simulink model "Control_Logic_a"  (R2018b)
settings: Solver=VariableStepAuto  StartTime=Start_time  StopTime=Stop_time  RelTol=1e-3
values from neighbouring files (symbols this model uses):
  Aset_N1 = 2    [Parameter_control.m]
  Aset_N10 = -10    [Parameter_control.m]
  Aset_N11 = 10    [Parameter_control.m]
  Aset_N12 = 20    [Parameter_control.m]
  Aset_N13 = 20    [Parameter_control.m]
  Aset_N2 = 30    [Parameter_control.m]
  Aset_N3 = 3    [Parameter_control.m]
  Aset_N4 = 5    [Parameter_control.m]
  Aset_N5 = 1    [Parameter_control.m]
  Aset_N6 = 0    [Parameter_control.m]
  Aset_N7 = 0.01    [Parameter_control.m]
  Aset_N8 = 2    [Parameter_control.m]
  Aset_N9 = 0.1    [Parameter_control.m]
  Dset_N1 = 1    [Parameter_control.m]
  Dset_N2 = 1    [Parameter_control.m]
  Ini_time = Start_time    (= 0)    [main.m]
  Sample_time = 0.1    [main.m]    (also in manual_env_for_test_slx.m; test_tool_initialize.m)
undefined symbols (not defined in the file or in its folder): DiscIntNeverNeededParam
(part 2 of 2)

== system Control_Logic_a/OST7 ==
  In : Inport  OutDataTypeStr=boolean  SampleTime=Sample_time
  T : Inport  Port=2  OutDataTypeStr=double  SampleTime=Sample_time
  Add : Sum  OutDataTypeStr=double
  Constant1 : Constant  SampleTime=Sample_time
  Discrete-Time Integrator1 : DiscreteIntegrator  SampleTime=Sample_time  LimitOutput=on  LowerSaturationLimit=0  ICPrevOutput=DiscIntNeverNeededParam  ICPrevScaledInput=DiscIntNeverNeededParam
  Logical Operator1 : Logic  AllPortsSameDT=off  OutDataTypeStr=boolean
  Max : MinMax  Inputs=2  OutDataTypeStr=double
  Parameter : Constant  Value=0  OutDataTypeStr=double  SampleTime=Sample_time
  Relational Operator : RelationalOperator  Operator=>  OutDataTypeStr=boolean  RndMeth=Nearest
  Sub : Sum  Inputs=+-  AccumDataTypeStr=single  OutDataTypeStr=double
  Switch : Switch  Criteria=u2 > Threshold  Threshold=0.5  OutDataTypeStr=double
  Unit Delay : UnitDelay  SampleTime=Sample_time
  Unit Delay2 : UnitDelay  InitialCondition=Ini_time  SampleTime=Sample_time
  Out : Outport  OutDataTypeStr=boolean  SampleTime=Sample_time
  wires:
  Constant1/1 -> Discrete-Time Integrator1/1
  Max/1 -> Relational Operator/2, Unit Delay/1
  T/1 -> Max/1, Relational Operator/1
  Add/1 -> Max/2
  Parameter/1 -> Switch/3
  Unit Delay/1 -> Switch/1
  Switch/1 -> Add/2
  Relational Operator/1 -> Logical Operator1/1
  Logical Operator1/1 -> Out/1
  Sub/1 -> Add/1
  Unit Delay2/1 -> Sub/2
  Discrete-Time Integrator1/1 -> Sub/1, Unit Delay2/1
  In/1 -> Logical Operator1/2, Switch/2

== system Control_Logic_a/OST8 ==
  In : Inport  OutDataTypeStr=boolean  SampleTime=Sample_time
  T : Inport  Port=2  OutDataTypeStr=double  SampleTime=Sample_time
  Add : Sum  OutDataTypeStr=double
  Constant1 : Constant  SampleTime=Sample_time
  Discrete-Time Integrator1 : DiscreteIntegrator  SampleTime=Sample_time  LimitOutput=on  LowerSaturationLimit=0  ICPrevOutput=DiscIntNeverNeededParam  ICPrevScaledInput=DiscIntNeverNeededParam
  Logical Operator1 : Logic  AllPortsSameDT=off  OutDataTypeStr=boolean
  Max : MinMax  Inputs=2  OutDataTypeStr=double
  Parameter : Constant  Value=0  OutDataTypeStr=double  SampleTime=Sample_time
  Relational Operator : RelationalOperator  Operator=>  OutDataTypeStr=boolean  RndMeth=Nearest
  Sub : Sum  Inputs=+-  AccumDataTypeStr=single  OutDataTypeStr=double
  Switch : Switch  Criteria=u2 > Threshold  Threshold=0.5  OutDataTypeStr=double
  Unit Delay : UnitDelay  SampleTime=Sample_time
  Unit Delay2 : UnitDelay  InitialCondition=Ini_time  SampleTime=Sample_time
  Out : Outport  OutDataTypeStr=boolean  SampleTime=Sample_time
  wires:
  Constant1/1 -> Discrete-Time Integrator1/1
  Max/1 -> Relational Operator/2, Unit Delay/1
  T/1 -> Max/1, Relational Operator/1
  Add/1 -> Max/2
  Parameter/1 -> Switch/3
  Unit Delay/1 -> Switch/1
  Switch/1 -> Add/2
  Relational Operator/1 -> Logical Operator1/1
  Logical Operator1/1 -> Out/1
  Sub/1 -> Add/1
  Unit Delay2/1 -> Sub/2
  Discrete-Time Integrator1/1 -> Sub/1, Unit Delay2/1
  In/1 -> Logical Operator1/2, Switch/2

== system Control_Logic_a/OST9 ==
  In : Inport  OutDataTypeStr=boolean  SampleTime=Sample_time
  T : Inport  Port=2  OutDataTypeStr=double  SampleTime=Sample_time
  Add : Sum  OutDataTypeStr=double
  Constant1 : Constant  SampleTime=Sample_time
  Discrete-Time Integrator1 : DiscreteIntegrator  SampleTime=Sample_time  LimitOutput=on  LowerSaturationLimit=0  ICPrevOutput=DiscIntNeverNeededParam  ICPrevScaledInput=DiscIntNeverNeededParam
  Logical Operator1 : Logic  AllPortsSameDT=off  OutDataTypeStr=boolean
  Max : MinMax  Inputs=2  OutDataTypeStr=double
  Parameter : Constant  Value=0  OutDataTypeStr=double  SampleTime=Sample_time
  Relational Operator : RelationalOperator  Operator=>  OutDataTypeStr=boolean  RndMeth=Nearest
  Sub : Sum  Inputs=+-  AccumDataTypeStr=single  OutDataTypeStr=double
  Switch : Switch  Criteria=u2 > Threshold  Threshold=0.5  OutDataTypeStr=double
  Unit Delay : UnitDelay  SampleTime=Sample_time
  Unit Delay2 : UnitDelay  InitialCondition=Ini_time  SampleTime=Sample_time
  Out : Outport  OutDataTypeStr=boolean  SampleTime=Sample_time
  wires:
  Constant1/1 -> Discrete-Time Integrator1/1
  In/1 -> Switch/2, Logical Operator1/2
  Discrete-Time Integrator1/1 -> Unit Delay2/1, Sub/1
  Unit Delay2/1 -> Sub/2
  Sub/1 -> Add/1
  Logical Operator1/1 -> Out/1
  Relational Operator/1 -> Logical Operator1/1
  Switch/1 -> Add/2
  Unit Delay/1 -> Switch/1
  Parameter/1 -> Switch/3
  Add/1 -> Max/2
  T/1 -> Relational Operator/1, Max/1
  Max/1 -> Unit Delay/1, Relational Operator/2

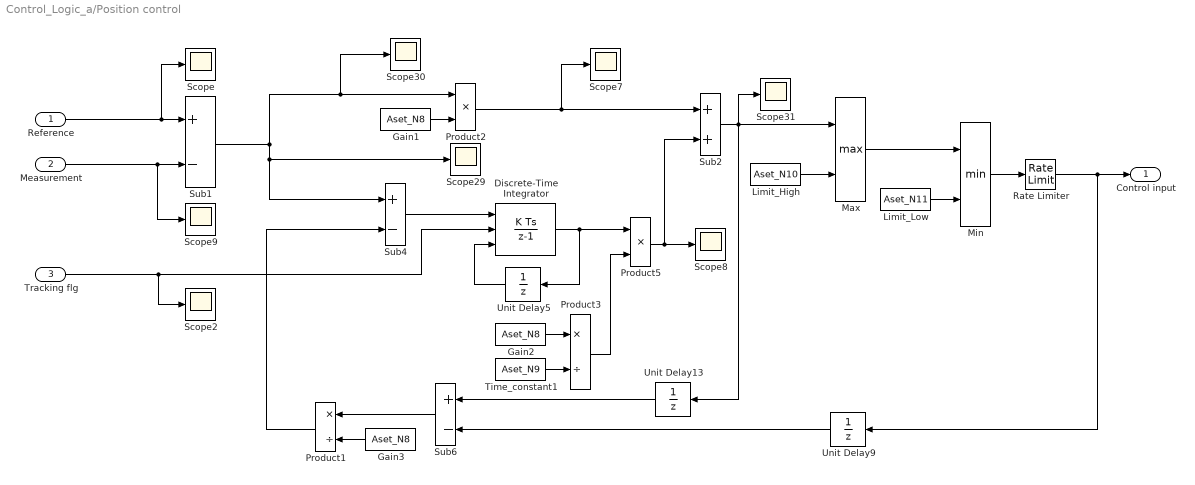
== system Control_Logic_a/Position control ==
  Reference : Inport
  Measurement : Inport  Port=2
  Tracking flg : Inport  Port=3
  Discrete-Time Integrator : DiscreteIntegrator  ExternalReset=level  InitialConditionSource=external  SampleTime=Sample_time  ICPrevOutput=DiscIntNeverNeededParam  ICPrevScaledInput=DiscIntNeverNeededParam
  Gain1 : Constant  Value=Aset_N8  OutDataTypeStr=double  SampleTime=Sample_time
  Gain2 : Constant  Value=Aset_N8  OutDataTypeStr=double  SampleTime=Sample_time
  Gain3 : Constant  Value=Aset_N8  OutDataTypeStr=double  SampleTime=Sample_time
  Limit_High : Constant  Value=Aset_N10  OutDataTypeStr=double  SampleTime=Sample_time
  Limit_Low : Constant  Value=Aset_N11  OutDataTypeStr=double  SampleTime=Sample_time
  Max : MinMax  Function=max  Inputs=2
  Min : MinMax  Inputs=2
  Product1 : Product  Inputs=*/  OutDataTypeStr=double  RndMeth=Zero
  Product2 : Product  OutDataTypeStr=double  RndMeth=Zero
  Product3 : Product  Inputs=*/  OutDataTypeStr=double  RndMeth=Zero
  Product5 : Product  Inputs=**  OutDataTypeStr=double  RndMeth=Zero
  Rate Limiter : RateLimiter  RisingSlewLimit=Aset_N12  FallingSlewLimit=-1*Aset_N13  SampleTimeMode=inherited
  Scope{,2,7..9,29..31} (8 alike) : Scope
  Sub1 : Sum  Inputs=+-  OutDataTypeStr=double
  Sub2 : Sum  OutDataTypeStr=double
  Sub4 : Sum  Inputs=+-  OutDataTypeStr=double
  Sub6 : Sum  Inputs=+-  OutDataTypeStr=double
  Time_constant1 : Constant  Value=Aset_N9  OutDataTypeStr=double  SampleTime=Sample_time
  Unit Delay13 : UnitDelay  SampleTime=Sample_time
  Unit Delay5 : UnitDelay  SampleTime=Sample_time
  Unit Delay9 : UnitDelay  SampleTime=Sample_time
  Control input : Outport
  wires:
  Sub2/1 -> Unit Delay13/1, Scope31/1, Max/1
  Measurement/1 -> Scope9/1, Sub1/2
  Sub1/1 -> Scope30/1, Product2/1, Scope29/1, Sub4/1
  Product3/1 -> Product5/2
  Unit Delay13/1 -> Sub6/1
  Product2/1 -> Scope7/1, Sub2/1
  Sub6/1 -> Product1/1
  Sub4/1 -> Discrete-Time Integrator/1
  Gain1/1 -> Product2/2
  Min/1 -> Rate Limiter/1
  Reference/1 -> Scope/1, Sub1/1
  Gain3/1 -> Product1/2
  Limit_Low/1 -> Min/2
  Unit Delay5/1 -> Discrete-Time Integrator/3
  Tracking flg/1 -> Scope2/1, Discrete-Time Integrator/2
  Discrete-Time Integrator/1 -> Unit Delay5/1, Product5/1
  Limit_High/1 -> Max/2
  Product5/1 -> Scope8/1, Sub2/2
  Rate Limiter/1 -> Control input/1, Unit Delay9/1
  Time_constant1/1 -> Product3/2
  Gain2/1 -> Product3/1
  Max/1 -> Min/1
  Product1/1 -> Sub4/2
  Unit Delay9/1 -> Sub6/2

== system Control_Logic_a/SSR ==
  S : Inport
  R : Inport  Port=2
  Logical Operator1 : Logic  Operator=OR  AllPortsSameDT=off  OutDataTypeStr=boolean
  Logical Operator2 : Logic  AllPortsSameDT=off  OutDataTypeStr=boolean
  Logical Operator5 : Logic  Operator=NOT  AllPortsSameDT=off  OutDataTypeStr=boolean
  Unit Delay : UnitDelay  SampleTime=Sample_time
  Out : Outport
  wires:
  Logical Operator5/1 -> Logical Operator2/1
  R/1 -> Logical Operator5/1
  Unit Delay/1 -> Logical Operator2/2
  Logical Operator2/1 -> Logical Operator1/2
  Logical Operator1/1 -> Unit Delay/1, Out/1
  S/1 -> Logical Operator1/1

== system Control_Logic_a/SSR1 ==
  S : Inport
  R : Inport  Port=2
  Logical Operator1 : Logic  Operator=OR  AllPortsSameDT=off  OutDataTypeStr=boolean
  Logical Operator2 : Logic  AllPortsSameDT=off  OutDataTypeStr=boolean
  Logical Operator5 : Logic  Operator=NOT  AllPortsSameDT=off  OutDataTypeStr=boolean
  Unit Delay : UnitDelay  SampleTime=Sample_time
  Out : Outport
  wires:
  Logical Operator5/1 -> Logical Operator2/1
  R/1 -> Logical Operator5/1
  Unit Delay/1 -> Logical Operator2/2
  Logical Operator2/1 -> Logical Operator1/2
  Logical Operator1/1 -> Unit Delay/1, Out/1
  S/1 -> Logical Operator1/1

== system Control_Logic_a/SSR2 ==
  S : Inport
  R : Inport  Port=2
  Logical Operator1 : Logic  Operator=OR  AllPortsSameDT=off  OutDataTypeStr=boolean
  Logical Operator2 : Logic  AllPortsSameDT=off  OutDataTypeStr=boolean
  Logical Operator5 : Logic  Operator=NOT  AllPortsSameDT=off  OutDataTypeStr=boolean
  Unit Delay : UnitDelay  SampleTime=Sample_time
  Out : Outport
  wires:
  S/1 -> Logical Operator1/1
  Logical Operator1/1 -> Out/1, Unit Delay/1
  Logical Operator2/1 -> Logical Operator1/2
  Unit Delay/1 -> Logical Operator2/2
  R/1 -> Logical Operator5/1
  Logical Operator5/1 -> Logical Operator2/1

== system Control_Logic_a/SSR3 ==
  S : Inport
  R : Inport  Port=2
  Logical Operator1 : Logic  Operator=OR  AllPortsSameDT=off  OutDataTypeStr=boolean
  Logical Operator2 : Logic  AllPortsSameDT=off  OutDataTypeStr=boolean
  Logical Operator5 : Logic  Operator=NOT  AllPortsSameDT=off  OutDataTypeStr=boolean
  Unit Delay : UnitDelay  SampleTime=Sample_time
  Out : Outport
  wires:
  Logical Operator5/1 -> Logical Operator2/1
  R/1 -> Logical Operator5/1
  Unit Delay/1 -> Logical Operator2/2
  Logical Operator2/1 -> Logical Operator1/2
  Logical Operator1/1 -> Unit Delay/1, Out/1
  S/1 -> Logical Operator1/1

== system Control_Logic_a/SSR4 ==
  S : Inport
  R : Inport  Port=2
  Logical Operator1 : Logic  Operator=OR  AllPortsSameDT=off  OutDataTypeStr=boolean
  Logical Operator2 : Logic  AllPortsSameDT=off  OutDataTypeStr=boolean
  Logical Operator5 : Logic  Operator=NOT  AllPortsSameDT=off  OutDataTypeStr=boolean
  Unit Delay : UnitDelay  SampleTime=Sample_time
  Out : Outport
  wires:
  S/1 -> Logical Operator1/1
  Logical Operator1/1 -> Out/1, Unit Delay/1
  Logical Operator2/1 -> Logical Operator1/2
  Unit Delay/1 -> Logical Operator2/2
  R/1 -> Logical Operator5/1
  Logical Operator5/1 -> Logical Operator2/1

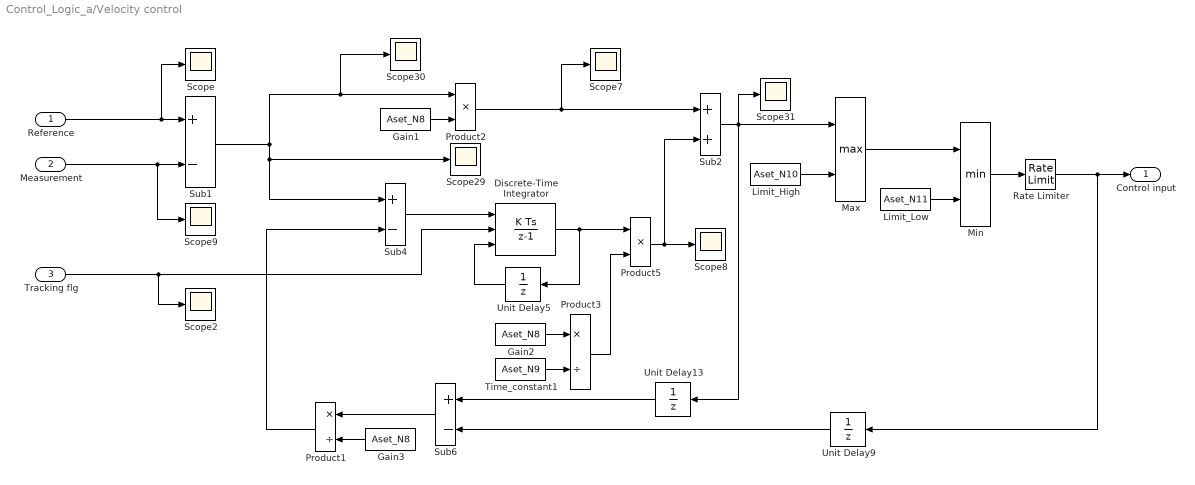
== system Control_Logic_a/Velocity control ==
  Reference : Inport
  Measurement : Inport  Port=2
  Tracking flg : Inport  Port=3
  Discrete-Time Integrator : DiscreteIntegrator  ExternalReset=level  InitialConditionSource=external  SampleTime=Sample_time  ICPrevOutput=DiscIntNeverNeededParam  ICPrevScaledInput=DiscIntNeverNeededParam
  Gain1 : Constant  Value=Aset_N8  OutDataTypeStr=double  SampleTime=Sample_time
  Gain2 : Constant  Value=Aset_N8  OutDataTypeStr=double  SampleTime=Sample_time
  Gain3 : Constant  Value=Aset_N8  OutDataTypeStr=double  SampleTime=Sample_time
  Limit_High : Constant  Value=Aset_N10  OutDataTypeStr=double  SampleTime=Sample_time
  Limit_Low : Constant  Value=Aset_N11  OutDataTypeStr=double  SampleTime=Sample_time
  Max : MinMax  Function=max  Inputs=2
  Min : MinMax  Inputs=2
  Product1 : Product  Inputs=*/  OutDataTypeStr=double  RndMeth=Zero
  Product2 : Product  OutDataTypeStr=double  RndMeth=Zero
  Product3 : Product  Inputs=*/  OutDataTypeStr=double  RndMeth=Zero
  Product5 : Product  Inputs=**  OutDataTypeStr=double  RndMeth=Zero
  Rate Limiter : RateLimiter  RisingSlewLimit=Aset_N12  FallingSlewLimit=-1*Aset_N13  SampleTimeMode=inherited
  Scope{,2,7..9,29..31} (8 alike) : Scope
  Sub1 : Sum  Inputs=+-  OutDataTypeStr=double
  Sub2 : Sum  OutDataTypeStr=double
  Sub4 : Sum  Inputs=+-  OutDataTypeStr=double
  Sub6 : Sum  Inputs=+-  OutDataTypeStr=double
  Time_constant1 : Constant  Value=Aset_N9  OutDataTypeStr=double  SampleTime=Sample_time
  Unit Delay13 : UnitDelay  SampleTime=Sample_time
  Unit Delay5 : UnitDelay  SampleTime=Sample_time
  Unit Delay9 : UnitDelay  SampleTime=Sample_time
  Control input : Outport
  wires:
  Unit Delay9/1 -> Sub6/2
  Product1/1 -> Sub4/2
  Max/1 -> Min/1
  Gain2/1 -> Product3/1
  Time_constant1/1 -> Product3/2
  Rate Limiter/1 -> Unit Delay9/1, Control input/1
  Product5/1 -> Sub2/2, Scope8/1
  Limit_High/1 -> Max/2
  Discrete-Time Integrator/1 -> Product5/1, Unit Delay5/1
  Tracking flg/1 -> Discrete-Time Integrator/2, Scope2/1
  Unit Delay5/1 -> Discrete-Time Integrator/3
  Limit_Low/1 -> Min/2
  Gain3/1 -> Product1/2
  Reference/1 -> Sub1/1, Scope/1
  Min/1 -> Rate Limiter/1
  Gain1/1 -> Product2/2
  Sub4/1 -> Discrete-Time Integrator/1
  Sub6/1 -> Product1/1
  Product2/1 -> Sub2/1, Scope7/1
  Unit Delay13/1 -> Sub6/1
  Product3/1 -> Product5/2
  Sub1/1 -> Sub4/1, Scope29/1, Product2/1, Scope30/1
  Measurement/1 -> Sub1/2, Scope9/1
  Sub2/1 -> Max/1, Scope31/1, Unit Delay13/1
